simulink model "lab2_Q2_R2023a"  (R2023a)
settings: Solver=VariableStepAuto  StartTime=0.0  StopTime=5  RelTol=1e-3
libraries: spsSeriesRLCBranchLib x5, spsMosfetLib x4, spsVoltageMeasurementLib x2, spsCurrentMeasurementLib x1, spsPVArrayLib x1, spsPWMGeneratorDCDCLib x1, sps_lib x1
settings Model: Creator=andre  LastModifiedBy=andre

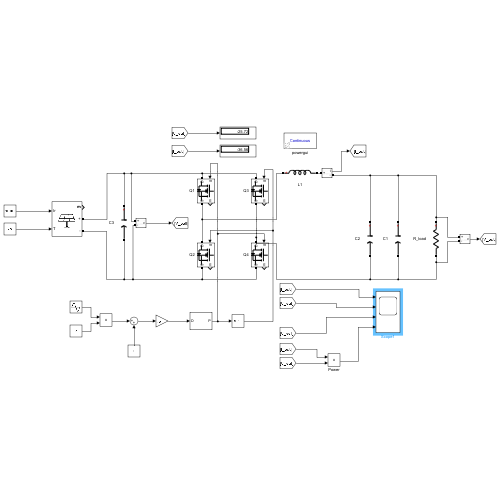
[thumbnail: Simulink's stored preview of the top-level diagram]
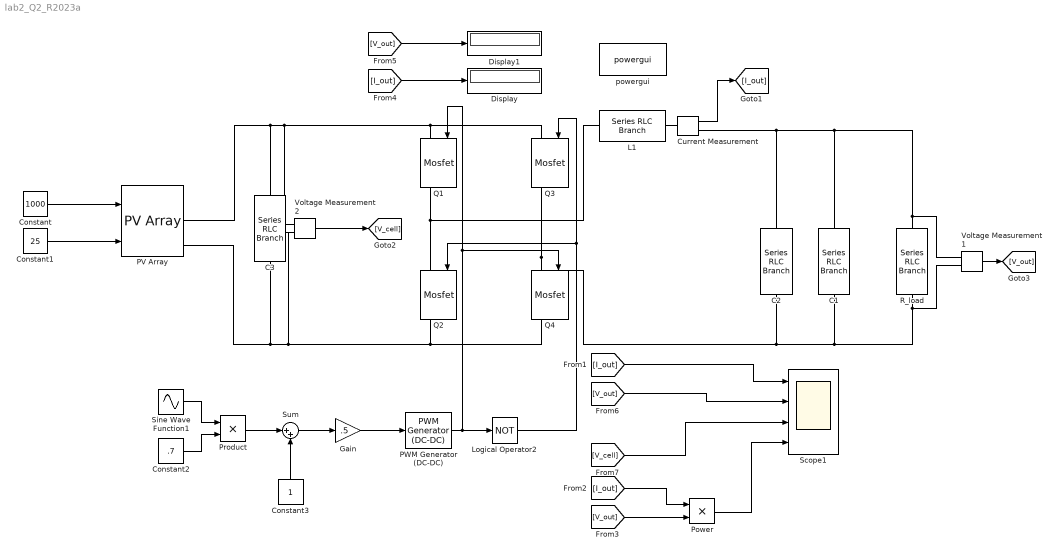
== system lab2_Q2_R2023a ==
  C1 : spsSeriesRLCBranchLib/Series RLC Branch  LConnTagsString=__new0  RConnTagsString=__new0  BranchType=C  Resistance=1  Inductance=1e-3  SetiL0=off  InitialCurrent=0  Capacitance=68e-6  Setx0=off  InitialVoltage=0  Measurements=None
  C2 : spsSeriesRLCBranchLib/Series RLC Branch  LConnTagsString=__new0  RConnTagsString=__new0  BranchType=C  Resistance=1  Inductance=1e-3  SetiL0=off  InitialCurrent=0  Capacitance=68e-6  Setx0=off  InitialVoltage=0  Measurements=None
  C3 : spsSeriesRLCBranchLib/Series RLC Branch  LConnTagsString=__new0  RConnTagsString=__new0  BranchType=C  Resistance=1  Inductance=1e-3  SetiL0=off  InitialCurrent=0  Capacitance=4e-3  Setx0=off  InitialVoltage=0  Measurements=None
  Constant : Constant  Value=1000
  Constant1 : Constant  Value=25
  Constant2 : Constant  Value=.7
  Constant3 : Constant
  Current Measurement : spsCurrentMeasurementLib/Current Measurement  PhasorSimulation=off  OutputType=Complex  PSBequivalent=0
  Display : Display
  Display1 : Display
  Gain : Gain  Gain=.5
  L1 : spsSeriesRLCBranchLib/Series RLC Branch  LConnTagsString=__new0  RConnTagsString=__new0  BranchType=L  Resistance=1  Inductance=520e-6  SetiL0=off  InitialCurrent=0  Capacitance=1e-6  Setx0=off  InitialVoltage=0  Measurements=None
  Logical Operator2 : Logic  Operator=NOT  AllPortsSameDT=off  OutDataTypeStr=boolean
  PV Array : spsPVArrayLib/PV Array  Npar=40  Nser=10  PlotType=array @ 1000 W/m2 & specified temperatures  S_vec="[ 1000  500  100 ]"  Temp_C_vec="[ 25  ]"  ModuleName=SolarWorld Industries GmbH Sunmodule Plus SW 250 mono black  PlotWhenSelected=off  Pm=250.355  Ncell=60  Voc=37.8  Isc=8.28  Vm=31.1  Im=8.05  beta_Voc_pc=-0.313  alpha_Isc_pc=0.005  beta_Voc=-0.11831  alpha_Isc=0.000414  IL=8.3819  I0=4.5375e-11  nI=0.94533  Rsh=1469.9171  Rs=0.28491  RobustModel=off  RobustCellTemperature=313.3991  BAL=on  Tc=1e-6  Tfilter=5e-5
  PWM Generator (DC-DC) : spsPWMGeneratorDCDCLib/PWM Generator (DC-DC)  Fsw=5000  Ts=0
  Power : Product
  Product : Product
  Q{1..4} (4 alike) : spsMosfetLib/Mosfet  Ron=0.1  Lon=0  Rd=0.01  Vfd=0  IC=0  Rs=1e5  Cs=inf  Measurements=on
  R_load : spsSeriesRLCBranchLib/Series RLC Branch  LConnTagsString=__new0  RConnTagsString=__new0  BranchType=R  Resistance=2  Inductance=1e-3  SetiL0=off  InitialCurrent=0  Capacitance=1e-6  Setx0=off  InitialVoltage=0  Measurements=None
  Scope1 : Scope  NumInputPorts=4
  Sine Wave Function1 : Sin  Frequency=2*pi*60  SampleTime=0
  Sum : Sum  Inputs=|++
  Voltage Measurement1 : spsVoltageMeasurementLib/Voltage Measurement  PhasorSimulation=off  OutputType=Complex  PSBequivalent=0
  Voltage Measurement2 : spsVoltageMeasurementLib/Voltage Measurement  PhasorSimulation=off  OutputType=Complex  PSBequivalent=0
  powergui : sps_lib/powergui  Priority=1  SimulationMode=Continuous  SampleTime=50e-6  frequency=60  Iterations=50  frequencyindice=0  Pbase=100e6  ErrMax=1e-4  UnitsV=kV  UnitsW=MW  buscounter=0  FunctionMessages=off  echomessages=off  EnableUseOfTLC=off  CurrentSourceSwitches=off  DisableSnubberDevices=off  DisableRonSwitches=off  DisableVfSwitches=off  DisplayEquations=off  AutomaticDiscreteSolvers=off  SolverType=Tustin/Backward Euler (TBE)  Interpol=off  ExternalGateDelay=off  methode=off  Ts=100  x0status=blocks  SPID=on  SwTol=0  HookPort=off  NonlinearTolerance=1e-4  nMaxIteration=100  ContinueOnMaxIteration=off  RestoreLinks=warning  ResistiveCurrentMeasurement=off  Frange=[0:2:500]  Ylog=off  Xlog=on  ShowGrid=off  save=off  variable=ZData  structure=0  ZoomFFT=off  StartTime=0.0  cycles=1  DisplayStyle=1  fundamental=60  FreqAxis=off  MaxFrequency=1000  frequencyindicesteady=1  RmsSteady=1  display=off
  wires:
  [I_out] -> Power/1
  [I_out] -> Display/1
  [V_out] -> Power/2
  Power/1 -> Scope1/4
  [V_out] -> Display1/1
  Current Measurement/1 -> [I_out]
  Voltage Measurement1/1 -> [V_out]
  [V_out] -> Scope1/2
  [I_out] -> Scope1/1
  Constant/1 -> PV Array/1
  Constant1/1 -> PV Array/2
  PWM Generator (DC-DC)/1 -> Logical Operator2/1, Q4/1, Q1/1
  Constant2/1 -> Product/2
  Product/1 -> Sum/1
  Sine Wave Function1/1 -> Product/1
  Sum/1 -> Gain/1
  Gain/1 -> PWM Generator (DC-DC)/1
  Constant3/1 -> Sum/2
  Logical Operator2/1 -> Q2/1, Q3/1
  Voltage Measurement2/1 -> [V_cell]
  [V_cell] -> Scope1/3
  connections:
  Q2/LConn1 -- Q1/RConn1 -- L1/LConn1
  Q4/RConn1 -- PV Array/RConn2 -- C3/RConn1 -- Voltage Measurement2/LConn2 -- Q2/RConn1
  R_load/LConn1 -- C2/LConn1 -- Current Measurement/RConn1 -- C1/LConn1 -- Voltage Measurement1/LConn1
  Q4/LConn1 -- C2/RConn1 -- Voltage Measurement1/LConn2 -- R_load/RConn1 -- C1/RConn1 -- Q3/RConn1
  Q1/LConn1 -- PV Array/RConn1 -- C3/LConn1 -- Voltage Measurement2/LConn1 -- Q3/LConn1
  Current Measurement/LConn1 -- L1/RConn1
